simulink model "Simulation05"  (R2018a)
settings: Solver=VariableStepAuto  StartTime=0.0  StopTime=100  RelTol=1e-3
libraries: simulink x2
settings Model: Creator=dasun  LastModifiedBy=dasun

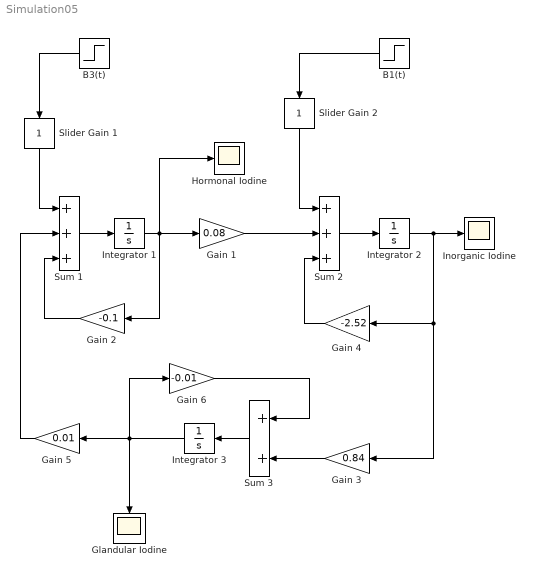
== system Simulation05 ==
  B1(t) : Step  Time=0  After=15  SampleTime=0
  B3(t) : Step  Time=0  After=0  SampleTime=0
  "Gain 1 " : Gain  Gain=0.08
  "Gain 2 " : Gain  Gain=-0.1
  "Gain 3 " : Gain  Gain=0.84
  "Gain 4 " : Gain  Gain=-2.52
  Gain 5 : Gain  Gain=0.01
  "Gain 6 " : Gain  Gain=-0.01
  Glandular Iodine : Scope
  Hormonal Iodine : Scope
  Inorganic Iodine : Scope
  "Integrator 1 " : Integrator  InitialCondition=682
  "Integrator 2 " : Integrator  InitialCondition=81.2
  Integrator 3 : Integrator  InitialCondition=6821
  Slider Gain 1 : simulink/Math Operations/Slider Gain  gain=1  low=0  high=2
  Slider Gain 2 : simulink/Math Operations/Slider Gain  gain=1  low=0  high=15
  Sum 1 : Sum  Inputs=+++
  "Sum 2 " : Sum  Inputs=+++
  Sum 3 : Sum
  wires:
  "Sum 2 "/1 -> "Integrator 2 "/1
  "Integrator 2 "/1 -> "Gain 4 "/1, "Gain 3 "/1, Inorganic Iodine/1
  B1(t)/1 -> Slider Gain 2/1
  Slider Gain 2/1 -> "Sum 2 "/1
  "Gain 1 "/1 -> "Sum 2 "/2
  "Integrator 1 "/1 -> "Gain 2 "/1, Hormonal Iodine/1, "Gain 1 "/1
  Sum 1/1 -> "Integrator 1 "/1
  B3(t)/1 -> Slider Gain 1/1
  "Gain 4 "/1 -> "Sum 2 "/3
  Sum 3/1 -> Integrator 3/1
  Integrator 3/1 -> Gain 5/1, "Gain 6 "/1, Glandular Iodine/1
  "Gain 3 "/1 -> Sum 3/2
  "Gain 6 "/1 -> Sum 3/1
  "Gain 2 "/1 -> Sum 1/3
  Gain 5/1 -> Sum 1/2
  Slider Gain 1/1 -> Sum 1/1
